simulink model "testemplannerglf_cs"  (R2020a)
settings: Solver=ode5  StartTime=0.0  StopTime=75  FixedStep=1/1000  RelTol=1e-3
PreLoadFcn:
  | mbxruntime.callbacks.PreLoadFcn(bdroot);
PostLoadFcn:
  | mbxruntime.callbacks.PostLoadFcn(bdroot);
InitFcn:
  | mbxruntime.callbacks.InitFcn(bdroot);
StartFcn:
  | mbxruntime.callbacks.StartFcn(bdroot);
StopFcn:
  | mbxruntime.callbacks.StopFcn(bdroot);
model workspace (MAT data in the model file):
  mbox_table : object (value not decoded)
  model_closed = 0
  sim_status = 0
values from neighbouring files (symbols this model uses):
  global_path_x = [-3.342 -2.8421723782 -2.34265574205 -1.8434543045 -1.34457058078 -0.846006057582 -0.347761597731 0.15016231435 0.647765423738 1.14504761469 1.64200885585 2.13864916705 ... (1501 elements, 1501x1)]    [global_path.mat]
  global_path_y = [4.7606 4.76495870158 4.76931469124 4.77366793224 4.77801840264 4.78236608949 4.78671098525 4.7910530857 4.79539238863 4.79972889301 4.80406259858 4.80839350551 ... (1501 elements, 1501x1)]    [global_path.mat]
undefined symbols (not defined in the file or in its folder): DiscIntNeverNeededParam, warningInitialVelocity, x0
libraries: simulink x19, PreScanSimulinkLibrary x11, simulink_extras x6, Solver_SF x1
(part 6 of 7)

== matlab function testemplannerglf_cs/Audi_A8_Sedan_1/decesion&&planning/referenceline provider/calc_heading_kappa1 ==
  data: path_x input; frenet_heading output; path_y input; frenet_kappa output
function [frenet_heading,frenet_kappa] = fcn(path_x,path_y)
%功能：该函数是利用已知的路径点计算heading和Kappa的值
%输入：path_x，path_y，全局路径点
%输出：frenet_heading，kappa
%2022 0310 glf 于寝室302

%注意事项，这里要注意角度的多值性，
%计算kappa时，kappa = dheading/ds，如果dheading差pi时tan值相等
%x和x+2pi往往代表同一个角度，但是（0.1-（-0.1））/ds和（0.1-（-0.1+2*pi））/ds差距较大
dx = diff(path_x);
dy = diff(path_y);

dx_pre = [dx(1);dx];
dx_after = [dx;dx(end)];
dx_final = (dx_pre + dx_after) / 2;

dy_pre = [dy(1);dy];
dy_after = [dy;dy(end)];
dy_final = (dy_pre + dy_after) / 2;

frenet_heading = atan2(dy_final,dx_final);

ds = sqrt(dx_final.^2 + dy_final.^2);
dheading = diff(frenet_heading);
dheading_pre = [dheading(1);dheading];
dheading_after = [dheading;dheading(end)];
dheading_final = (dheading_pre + dheading_after) / 2;

%为了防止dheading出现多了一个2pi的错误，假设真实的dheading较小，用sin（dheading）近似dheading
frenet_kappa = sin(dheading_final). / ds;

== matlab function testemplannerglf_cs/Audi_A8_Sedan_2/PathFollower_Preview_1/LateralController/Calculate delta steering error/eml_delta_steering_error ==
  data: v_x_vehicle input; v_x_vehicle_Min input; t_Preview_LatCtrl input; delta_steeringwheeltotal output; v_y_vehicle input; yawrate_vehicle input; CorneringStiffness_Tyres_Front input; CorneringStiffness_Tyres_Rear input; m_vehicle_total input; inertia_z_vehicle_total input; e_Lat input size=10; Pos_x_CoG_Vehicle input; wheelbase input; RefreshCounter parameter
function delta_steeringwheeltotal = eml_delta_steering_error(v_x_vehicle,v_x_vehicle_Min,t_Preview_LatCtrl,v_y_vehicle,yawrate_vehicle,CorneringStiffness_Tyres_Front,CorneringStiffness_Tyres_Rear,m_vehicle_total,inertia_z_vehicle_total,e_Lat,Pos_x_CoG_Vehicle,wheelbase,RefreshCounter)

delta_steeringwheeltotal = emlfcn_delta_steering_error(v_x_vehicle,v_x_vehicle_Min,t_Preview_LatCtrl,v_y_vehicle,yawrate_vehicle,CorneringStiffness_Tyres_Front,CorneringStiffness_Tyres_Rear,m_vehicle_total,inertia_z_vehicle_total,e_Lat,Pos_x_CoG_Vehicle,wheelbase,RefreshCounter);

% end function

== matlab function testemplannerglf_cs/Audi_A8_Sedan_1/decesion&&planning/emplanner planner/plan_start&&switch_trajectory ==
  data: pre_trajectory_x input; pre_trajectory_y input; pre_trajectory_heading input; pre_trajectory_kappa input; pre_trajectory_velocity input; pre_trajectory_accel input; pre_trajectory_time input; current_time input; host_x input; host_y input; host_heading_xy input; host_vx input; host_vy input; host_ax input; host_ay input; plan_start_x output; plan_start_y output; plan_start_heading output; plan_start_kappa output; plan_start_vx output; plan_start_vy output; plan_start_ax output; plan_start_ay output; plan_start_time output; switch_x output; switch_y output; switch_heading output; switch_kappa output; switch_speed output; switch_accel output; switch_time output
function [plan_start_x,plan_start_y,plan_start_heading,plan_start_kappa,plan_start_vx,plan_start_vy,plan_start_ax,plan_start_ay,plan_start_time,...
    switch_x,switch_y,switch_heading,switch_kappa,switch_speed,switch_accel,switch_time] = fcn(pre_trajectory_x,pre_trajectory_y,pre_trajectory_heading,...
    pre_trajectory_kappa,pre_trajectory_velocity,pre_trajectory_accel,pre_trajectory_time,current_time,host_x,host_y,host_heading_xy,host_vx,host_vy,host_ax,host_ay)
%功能:该函数将提供规划起点，拼接轨迹的消息
%输入：
%上个轨迹点的信息pre_trajectory_x,pre_trajectory_y,pre_trajectory_heading，pre_trajectory_kappa,pre_trajectory_velocity,pre_trajectory_accel,pre_trajectory_time
%现在的时间：current_time
%定位消息：host_x,host_y,host_heading_xy,host_vx,host_vy,host_ax,host_ay
%输出：
%规划轨迹的消息：plan_start_x,plan_start_y,plan_start_heading,plan_start_kappa,plan_start_vx,plan_start_vy,plan_start_ax,plan_start_ay,plan_start_time
%拼接轨迹的消息：switch_x,switch_y,switch_heading,switch_kappa,switch_speed,switch_accel,switch_time

%20220312 glf写于寝室302
%对拼接的轨迹初始化
n = 20;
switch_x = zeros(n,1);
switch_y = zeros(n,1);
switch_heading = zeros(n,1);
switch_kappa = zeros(n,1);
switch_speed = zeros(n,1);
switch_accel = zeros(n,1);
switch_time = ones(n,1) * -1;
persistent isFirstRun;
if isempty(isFirstRun)
    %代码首次运行
    isFirstRun = 0;
    %首次运行车辆的速度为0，因此不需要车辆动力学进行外推
    plan_start_x = host_x;
    plan_start_y = host_y;
    plan_start_heading = host_heading_xy;
    plan_start_kappa = 0;
    plan_start_vx = 0;
    plan_start_vy = 0;
    plan_start_ax = 0;
    plan_start_ay = 0;
    plan_start_time = current_time+0.1;
else
    x_cur = host_x;
    y_cur = host_y;
    kappa_cur = 0;
    %将车辆坐标的速度转换为世界坐标系
    vx_cur = host_vx*cos(host_heading_xy) - host_vy*sin(host_heading_xy);
    vy_cur = host_vx*sin(host_heading_xy) + host_vy*cos(host_heading_xy);
    ax_cur = host_ax*cos(host_heading_xy) - host_ay*sin(host_heading_xy);
    ay_cur = host_ax*sin(host_heading_xy) + host_ay*cos(host_heading_xy);
    %规划周期
    dt = 0.1;
    %判断当前时间在上个轨迹的那个位置
    for i = 1:(length(pre_trajectory_time) - 1)
       if pre_trajectory_time(i) <= current_time && pre_trajectory_time(i+1) > current_time 
          break; 
       end
    end
    
    %计算横纵向误差判断控制是否控制的完美
    pre_desire_heading = pre_trajectory_heading(i);
    %切向量
    tor = [cos(pre_desire_heading);sin(pre_desire_heading)];
    %法向量
    nor = [-sin(pre_desire_heading);cos(pre_desire_heading)];
    %位失
    direction = [host_x;host_y] - [pre_trajectory_x(i);pre_trajectory_y(i)];
    %横向误差
    lat_err = abs(direction'*nor);
    %纵向误差
    lon_err = abs(direction'*tor);
    if (lon_err > 2.5 || lat_err > 0.5)
        %控制没跟上
        plan_start_x = x_cur + vx_cur*dt + 0.5*ax_cur*dt*dt;
        plan_start_y = y_cur + vy_cur*dt + 0.5*ay_cur*dt*dt;
        plan_start_vx = vx_cur + ax_cur * dt;
        plan_start_vy = vy_cur + ay_cur * dt;
        plan_start_ax = ax_cur;
        plan_start_ay = ay_cur;
        plan_start_heading = atan2(plan_start_vy,plan_start_vx);
        plan_start_kappa = kappa_cur;
        %规划起点是当前时间点+100ms
        plan_start_time = current_time + 0.1;
    else
        %控制能跟上
        for j = i:length(pre_trajectory_time)-1
           if pre_trajectory_time(j) <= current_time + 0.1 &&pre_trajectory_time(j+1) < current_time
              break; 
           end
        end
        plan_start_x = pre_trajectory_x(j);
        plan_start_y = pre_trajectory_y(j);
        plan_start_heading = pre_trajectory_heading(j);
        plan_start_kappa = pre_trajectory_kappa(j);
        plan_start_vx = pre_trajectory_velocity*cos(plan_start_heading);
        plan_start_vy = pre_trajectory_velocity*sin(plan_start_heading);
        %切向量和法向量
        tor = [cos(plan_start_heading);sin(plan_start_heading)];
        nor = [-sin(plan_start_heading);cos(plan_start_heading)];
        a_tor = pre_trajectory_accel(j)*tor;
        a_nor = pre_trajectory_velocity(j)^2*plan_start_kappa*nor;
        plan_start_ax = a_tor(1) + a_nor(1);
        plan_start_ay = a_tor(2) + a_nor(2);
        plan_start_time = pre_trajectory_time(j);
        
        %进行轨迹拼接
        %还有一个细节需要考虑，pre_trajectory x(j) y(j)...是规划的起点，那么在轨迹拼接时
        %需不需要在stitch_trajectory中把pre_trajectory x(j) y(j)...包含进去
        %答案是否定的，不应该包含进去，因为规划的起点在规划模块计算完成后的结果中包含，如果在拼接的时候
        %还要包含，那就等于规划起点包含了两次
        %除非本周期计算的轨迹不包含规划起点，那么stitch_trajectory可以包含规划起点
        %如果本周期计算的轨迹包含规划起点，那么stitch_trajectory不可以包含规划起点
        %我们选择规划包含起点，拼接不包含起点的做法
 
        %把起点去掉
        j = j - 1;
        if j > 19
            switch_x = pre_trajectory_x(j-19:j);
            switch_y = pre_trajectory_y(j-19:j);
            switch_heading = pre_trajectory_heading(j-19:j);
            switch_kappa = pre_trajectory_kappa(j-19:j);
            switch_speed = pre_trajectory_velocity(j-19:j);
            switch_accel = pre_trajectory_accel(j-19:j);
            switch_time = pre_trajectory_time(j-19:j);
            
        else
            switch_x(20-j+1:20) = pre_trajectory_x(1:j);
            switch_y(20-j+1:20) = pre_trajectory_y(1:j);
            switch_heading(20-j+1:20) = pre_trajectory_heading(1:j);
            switch_kappa(20-j+1:20) = pre_trajectory_kappa(1:j);
            switch_speed(20-j+1:20) = pre_trajectory_velocity(1:j);
            switch_accel(20-j+1:20) = pre_trajectory_accel(1:j);
            switch_time(20-j+1:20) = pre_trajectory_time(1:j);
        end
    end
end

== matlab function testemplannerglf_cs/Audi_A8_Sedan_1/decesion&&planning/emplanner planner/index2s_calc ==
  data: reference_x input; index2s output; reference_y input; origin_x input; origin_y input; origin_match_point_index input
function index2s = fcn(reference_x,reference_y,origin_x,origin_y,origin_match_point_index)
    %功能：此函数是为了计算参考线上所有点的索引所对应的长度关系
    %输入：
    %参考线坐标：reference_x,reference_y
    %匹配点坐标：origin_x,origin_y，匹配点索引：origin_match_point_index
    %输出：
    %index2s储存了181个点的长度

    %2022 0315  glf 写于国实507
    n = 181;%一共有181个点
    index2s = zeros(n,1);
    for i = 2:181
       index2s(i) = sqrt((reference_x(i) - reference_x(i - 1))^2 + (reference_y(i) - reference_y(i - 1))^2) + index2s(i-1); 
    end

    %将index2s转换为以投影点为坐标原点
    s0 = fcn1(index2s,reference_x,reference_y,origin_x,origin_y,origin_match_point_index);

    index2s = index2s - s0*ones(n,1);
end

function s = fcn1(index2s,reference_x,reference_y,proj_x,proj_y,proj_match_point_index)
    %判断投影点是在匹配点的前面还是后面
    vector_1 = [proj_x;proj_y] - [reference_x(proj_match_point_index);reference_y(proj_match_point_index)];
    if proj_match_point_index < length(reference_x)
        vector_2 = [reference_x(proj_match_point_index + 1);reference_y(proj_match_point_index + 1)] - [reference_x(proj_match_point_index);reference_y(proj_match_point_index)];
    else
        vector_2 = [reference_x(proj_match_point_index);reference_y(proj_match_point_index)] - [reference_x(proj_match_point_index - 1);reference_y(proj_match_point_index - 1)];
    end

    if vector_1' * vector_2 > 0
        %投影点在匹配点前边
        s = index2s(proj_match_point_index) + sqrt(vector_1' * vector_1);
    else
        %投影点在匹配点后边
        s = index2s(proj_match_point_index) - sqrt(vector_1' * vector_1);
    end

end

== matlab function testemplannerglf_cs/Audi_A8_Sedan_1/peception_module/MATLAB Function ==
  data: host_x input; obs_x_set_gcs output; host_y input; host_heading_xy input; obs_range input; obs_theta input; obs_velocity input; obs_velocity_heading input; obs_y_set_gcs output; obs_velocity_set_gcs output; obs_heading_set_gcs output
function [obs_x_set_gcs, obs_y_set_gcs, obs_velocity_set_gcs, obs_heading_set_gcs] = ...
    fcn(host_x, host_y, host_heading_xy, obs_range, obs_theta, obs_velocity, obs_velocity_heading)
%gcs 全局坐标系global coordinate system
%该函数是感知模块，输出障碍物的位置，速度大小，速度方向与世界坐标系x轴的夹角
%输入：定位信息host_x,host_y,host_heading_xy世界坐标系
%      障碍物在传感器坐标下的极坐标range，theta
%      障碍物的速度大小 velocity
%      障碍物的速度方向与x轴的夹角heading
%输出：障碍物在世界坐标系下的坐标x y v x与x轴的夹角heading
%      注意输出的heading是在障碍物的速度heading，不是障碍物的几何2heading

%传感器最多输出32个障碍物信息，但是事先不知道有多少个障碍物，需要做个缓存

%输出初始化
obs_x_set_gcs = ones(32,1) * nan;
obs_y_set_gcs = ones(32,1) * nan;
obs_velocity_set_gcs = ones(32,1) * nan;
obs_heading_set_gcs = ones(32,1) * nan;
%传感器极坐标的角度顺时针为正，世界坐标是逆时针为正
theta_transfer = -obs_theta * pi /180;
%velocity的方向是向北为0度，世界坐标系是以向东为0度
heading_transfer = (-obs_velocity_heading + 90 * ones(32,1)) * pi / 180;
%计算障碍物到传感器的x方向距离，y方向距离
x_transfer = obs_range.*cos(theta_transfer + host_heading_xy);
y_transfer = obs_range.*sin(theta_transfer + host_heading_xy);

%计算障碍物的世界坐标
for i = 1:32
    if obs_range(i) ~= 0
        obs_x_set_gcs(i) = x_transfer(i) + host_x + 2.17 * cos(host_heading_xy);
        obs_y_set_gcs(i) = y_transfer(i) + host_y + 2.17 * sin(host_heading_xy);
        obs_heading_set_gcs(i) = heading_transfer(i);
        obs_velocity_set_gcs(i) = obs_velocity(i);
    end
end

== matlab function testemplannerglf_cs/Audi_A8_Sedan_1/decesion&&planning/emplanner planner/start_project ==
  data: host_x input; match_point_index_set output; host_y input; frenet_x input; frenet_y input; frenet_heading input; frenet_kappa input; project_x_set output; project_y_set output; project_heading_set output; project_kappa_set output
function [match_point_index_set,project_x_set,project_y_set,project_heading_set,project_kappa_set] =...
    fcn(host_x,host_y,frenet_x,frenet_y,frenet_heading,frenet_kappa)
%功能：该函数是为了求投影点的x，y,heading,kappa值，其中分成了首次运行和非首次运行，非首次运行条件下可以利用上一个周期运行的结果加速运算
%输入：host_x,host_y,frenet_x,frenet_y,frenet_heading,frenet_kappa
%输出：match_point_index_set, project_x、y_set， project_heading_set,proj_kappa_set
%2022 0309 glf写于国实507

%输出初始化
n = 128;%128只是用来存储数据的，实际中只用了第一个点.之后可以试试如果n=1看看程序能不能运行！！！！！
match_point_index_set = ones(n,1) * nan;
project_x_set = ones(n,1) * nan;
project_y_set = ones(n,1) * nan;
project_heading_set = ones(n,1) * nan;
project_kappa_set = ones(n,1) * nan;

%声明持久变量
persistent isFirstRun;
persistent pre_match_point_index_set;
persistent pre_frenet_x_set;
persistent pre_frenet_y_set;
persistent pre_frenet_heading_set;
persistent pre_frenet_kappa_set;

if isempty(isFirstRun)
    isFirstRun = 0;
    pre_frenet_x_set = frenet_x;
    pre_frenet_y_set = frenet_y;
    pre_frenet_heading_set = frenet_heading;
    pre_frenet_kappa_set = frenet_kappa;
    %初始化match_point的结果
    pre_match_point_index_set = ones(n,1)*nan;
    
    for i = 1:length(host_x)
        if isnan(host_x(i))
           break; 
        end
        start_index = 1;
        min_distance = inf;
        increase_count = 0;
        for j = start_index:length(frenet_x)
            distance = sqrt((host_x(i) - frenet_x(j))^2 + (host_y(i) - frenet_y(j))^2);
            if distance < min_distance
               distance = min_distance;
               match_point_index_set(i) = j;
            else
                increase_count = increase_count + 1;
            end
            if increase_count == 50
               break; 
            end
        end
        
        %由匹配点求投影点
        match_point_index = match_point_index_set(i);
        match_point_index_x = pre_frenet_x_set(match_point_index);%这里源代码写的是frenet_path_x
        match_point_index_y = pre_frenet_y_set(match_point_index);
        %匹配点位失
        match_point_direction = [match_point_index_x;match_point_index_y];
        %带投影点位失
        host_direction = [host_x;host_y];
        match_point_index_heading = pre_frenet_heading_set(match_point_index);
        match_point_index_kappa = pre_frenet_kappa_set(match_point_index);
        ds = (host_direction - match_point_direction)'*[cos(match_point_index_heading);sin(match_point_index_heading)];
        proj_index_set = match_point_direction + ds*[cos(match_point_index_heading);sin(match_point_index_heading)];
        proj_index_heading = match_point_index_heading + ds * match_point_index_kappa;
        proj_index_kappa = match_point_index_kappa;
        
        %输出计算结果
        project_x_set(i) = proj_index_set(1);
        project_y_set(i) = proj_index_set(2);
        project_heading_set(i) = proj_index_heading;
        project_kappa_set(i) = proj_index_kappa;   
    end
    pre_match_point_index_set = match_point_index_set;
    
else
    for i = 1:length(host_x)
        
        start_index = pre_match_point_index_set(i);
        %以下判断语句是为了防止感知时出现bug，具体还不懂
        %声明increase_count_limit
        increase_count_limit = 5;
        if isnan(start_search_index)
            increase_count_limit = 50;
            %搜索起点设为1
            start_search_index = 1;            
        end
        increase_count = 0; 
        
        %由上一个匹配点计算车辆的行驶方向
        %匹配点位失
        vector_match_point_index = [pre_frenet_x_set(start_index);pre_frenet_y_set(start_index)];
        %待投影点位失
        vector_host_point_index = [host_x;host_y];
        match_point_index_heading = pre_frenet_heading_set(start_index);
        flag = (vector_host_point_index - vector_match_point_index)'*[cos(match_point_index_heading);sin(match_point_index_heading)];
        if flag > 0.001
            min_distance = inf;
            for j = start_index:length(frenet_x)
                distance = sqrt((host_x(i) - frenet_x(j))^2 + (host_y(i) - frenet_y(j))^2);
                if distance < min_distance
                   distance = min_distance;
                   match_point_index_set(i) = j;
                else
                    increase_count = increase_count + 1;
                end
                if increase_count == increase_count_limit
                   break; 
                end
            end
        elseif flag < -0.001
            min_distance = inf;
            for j = start_index:-1:1
                distance = sqrt((host_x(i) - frenet_x(j))^2 + (host_y(i) - frenet_y(j))^2);
                if distance < min_distance
                   distance = min_distance;
                   match_point_index_set(i) = j;
                else
                    increase_count = increase_count + 1;
                end
                if increase_count == increase_count_limit
                   break; 
                end
            end
        else
            match_point_index_set(i) = start_index;
        end
        
        %由匹配点求投影点
        match_point_index = match_point_index_set(i);
        match_point_index_x = pre_frenet_x_set(match_point_index);%这里源代码写的是frenet_path_x
        match_point_index_y = pre_frenet_y_set(match_point_index);
        %匹配点位失
        match_point_direction = [match_point_index_x;match_point_index_y];
        %带投影点位失
        host_direction = [host_x;host_y];
        match_point_index_heading = pre_frenet_heading_set(match_point_index);
        match_point_index_kappa = pre_frenet_kappa_set(match_point_index);
        ds = (host_direction - match_point_direction)'*[cos(match_point_index_heading);sin(match_point_index_heading)];
        proj_index_set = match_point_direction + ds*[cos(match_point_index_heading);sin(match_point_index_heading)];
        proj_index_heading = match_point_index_heading + ds * match_point_index_kappa;
        proj_index_kappa = match_point_index_kappa;
        
        %输出计算结果
        project_x_set(i) = proj_index_set(1);
        project_y_set(i) = proj_index_set(2);
        project_heading_set(i) = proj_index_heading;
        project_kappa_set(i) = proj_index_kappa; 
    end
    pre_frenet_x_set = frenet_x;
    pre_frenet_y_set = frenet_y;
    pre_frenet_heading_set = frenet_heading;
    pre_frenet_kappa_set = frenet_kappa;
    pre_match_point_index_set = match_point_index_set;
end

== matlab function testemplannerglf_cs/Audi_A8_Sedan_1/decesion&&planning/emplanner planner/cattesian2Frenet/s&&l_calc ==
  data: x_set input; s_set output; y_set input; frenet_x_set input; frenet_y_set input; proj_x_set input; proj_y_set input; proj_heading_set input; proj_match_point_index input; l_set output; index2s input
function [s_set,l_set] = fcn(x_set,y_set, frenet_x_set,frenet_y_set,proj_x_set,proj_y_set,proj_heading_set,proj_match_point_index,index2s)
%功能：该函数是将规划起点时投影点从世界坐标系转换为frenet坐标下的s、l
%输入：x_set,y_set:规划开始的点的x和y坐标
%     frenet_x_set,frenet_y_set参考线的x、y坐标
%     proj_heading_set投影点的航向角 proj_match_point_index ：投影点匹配点索引
%     index2s：s的索引和长度的关系,这种算法加速了计算速度缩短了时间
%输出：s_set，l_set：frenet坐标下的s和l坐标

%2022 0317   glf 写于国实507
    %输出初始化
    n = 128;
    s_set = ones(n,1)*nan;
    l_set = ones(n,1)*nan;
    for i = 1:length(x_set)
        if isnan(x_set(i))
           break; 
        end
        s_set(i) = clacSFromIndex2s(index2s,frenet_x_set,frenet_y_set,proj_x_set(i),proj_y_set(i),proj_match_point_index(i));
        n_r = [-sin(proj_heading_set(i));cos(proj_heading_set(i))];
        r_h = [x_set(i);y_set(i)];
        r_r = [proj_x_set(i);proj_y_set(i)];
        l_set(i) = (r_h - r_r)'*n_r;
    end
    
end
function s = clacSFromIndex2s(index2s,frenet_x_set,frenet_y_set,proj_x_set,proj_y_set,proj_match_point_index)
    %判断投影点是在匹配点的前面还是后面
    vector_1 = [proj_x_set;proj_y_set] - [frenet_x_set(proj_match_point_index);frenet_y_set(proj_match_point_index)];
    if proj_match_point_index < length(reference_x)
        vector_2 = [frenet_x_set(proj_match_point_index + 1);frenet_y_set(proj_match_point_index + 1)] - [frenet_x_set(proj_match_point_index);frenet_y_set(proj_match_point_index)];
    else
        vector_2 = [frenet_x_set(proj_match_point_index);frenet_y_set(proj_match_point_index)] - [frenet_x_set(proj_match_point_index - 1);frenet_y_set(proj_match_point_index - 1)];
    end

    if vector_1' * vector_2 > 0
        %投影点在匹配点前边
        s = index2s(proj_match_point_index) + sqrt(vector_1' * vector_1);
    else
        %投影点在匹配点后边
        s = index2s(proj_match_point_index) - sqrt(vector_1' * vector_1);
    end
end

== matlab function testemplannerglf_cs/Audi_A8_Sedan_1/decesion&&planning/emplanner planner/cattesian2Frenet/s_dot&&l_dot&&dl_calc ==
  data: l_set input; s_dot_set output; vx_set input; vy_set input; proj_heading_set input; proj_kappa_set input; l_dot_set output; dl_set output
function [s_dot_set,l_dot_set,dl_set] = fcn(l_set,vx_set,vy_set,proj_heading_set,proj_kappa_set)
%功能：此函数功能是为了计算由世界坐标系转换为极坐标系下的s_dot, l_dot, dl_set
%输入：l_set计算得到的l的坐标的集合
%      vx_set，vy_set：世界坐标系的速度
%      proj_heading_set投影点的航向角   proj_kappa_set投影点的曲率
%输出：s_dot_set,l_dot_set,dl_set 坐标转换后的结果

%2022 0317  glf  写于国实507
%输出初始化
n = 128;
s_dot_set = ones(n,1)*nan;
l_dot_set = ones(n,1)*nan;
dl_set = ones(n,1)*nan;

for i = 1:length(l_set)
    if isnan(l_set(i))
       break;
    end
    v_h = [vx_set(i);vy_set(i)];
    t_r = [cos(proj_heading_set(i));sin(proj_heading_set(i))];
    n_r = [-sin(proj_heading_set(i));cos(proj_heading_set(i))];
    s_dot_set(i) = v_h' * t_r / (1 - proj_kappa_set(i)*l_set(i));
    
    l_dot_set(i) = v_h' * n_r;
    
    %利用向量法计算dl要避免速度为0的情况
    if s_dot_set(i) == 0
       dl_set(i) = 0; 
    else
        dl_set(i) = l_dot_set(i)/s_dot_set(i);
    end
end

== matlab function testemplannerglf_cs/Audi_A8_Sedan_1/decesion&&planning/emplanner planner/cattesian2Frenet/s_dot2&&l_dot2&&ddl_set_calc ==
  data: s_dot_set input; s_dot2_set output; l_set input; dl_set input; proj_heading_set input; proj_kappa_set input; ax_set input; ay_set input; l_dot2_set output; ddl_set output
function [s_dot2_set,l_dot2_set,ddl_set] = fcn(s_dot_set,l_set,dl_set,proj_heading_set,proj_kappa_set,ax_set,ay_set)
%功能：该函数是为了计算世界坐标系转换为frenet坐标系条件下的s_dot2_set,l_dot2_set,ddl_set
%输入：s_dot_set：坐标转换后的s_dot
%      l_set：frenet坐标系中的l坐标
%      dl_set坐标转换后的dl
%      proj_heading_set，proj_kappa_set投影点的航向角和曲率
%      ax_set，ay_set车辆的加速度
%输出：转换后的坐标系s_dot2_set,l_dot2_set,ddl_set

%2022 0317   glf 写于国实507

%输出初始化
n = 128;
s_dot2_set = ones(n,1);
l_dot2_set = ones(n,1);
ddl_set = ones(n,1);

for i = 1:length(l_set)
   if isnan(l_set(i))
      break; 
   end
   a_h = [ax_set(i);ay_set(i)];
   t_r = [cos(proj_heading_set(i));sin(proj_heading_set(i))];
   n_r = [-sin(proj_heading_set(i));cos(proj_heading_set(i))];
   
   l_dot2_set(i) = a_h' * n_r - proj_kappa_set(i)*(1 - proj_kappa_set(i) * l_set(i)) * (s_dot_set^2);
   %这里将dkr/ds设置为0，因为这个值极小，设置为0可以简化运算
   s_dot2_set(i) = 1/(1 - proj_kappa_set(i) * l_set(i)) * (a_h' * t_r + 2 * proj_kappa_set(i) * s_dot_set(i)^2 * l_set(i));
   %利用向量法计算时会出现速度为0的情况，因此分情况讨论
   if abs(s_dot_set(i)) < 1e-6
       ddl_set(i) = 0;
   else
       ddl_set(i) = (l_dot2_set(i) - dl_set(i) * s_dot2_set)/(s_dot_set(i)^2);
   end
   
end

== matlab function testemplannerglf_cs/Audi_A8_Sedan_1/decesion&&planning/emplanner planner/static_obs_filter/obs_cartesian2Frenetj/s&&l_calc ==
  data: x_set input; s_set output; y_set input; frenet_x_set input; frenet_y_set input; proj_x_set input; proj_y_set input; proj_heading_set input; proj_match_point_index input; l_set output; index2s input
function [s_set,l_set] = fcn(x_set,y_set, frenet_x_set,frenet_y_set,proj_x_set,proj_y_set,proj_heading_set,proj_match_point_index,index2s)
%功能：该函数是将规划起点时投影点从世界坐标系转换为frenet坐标下的s、l
%输入：x_set,y_set:规划开始的点的x和y坐标
%     frenet_x_set,frenet_y_set参考线的x、y坐标
%     proj_heading_set投影点的航向角 proj_match_point_index ：投影点匹配点索引
%     index2s：s的索引和长度的关系,这种算法加速了计算速度缩短了时间
%输出：s_set，l_set：frenet坐标下的s和l坐标

%2022 0317   glf 写于国实507
    %输出初始化
    n = 128;
    s_set = ones(n,1)*nan;
    l_set = ones(n,1)*nan;
    for i = 1:length(x_set)
        if isnan(x_set(i))
           break; 
        end
        s_set(i) = clacSFromIndex2s(index2s,frenet_x_set,frenet_y_set,proj_x_set(i),proj_y_set(i),proj_match_point_index(i));
        n_r = [-sin(proj_heading_set(i));cos(proj_heading_set(i))];
        r_h = [x_set(i);y_set(i)];
        r_r = [proj_x_set(i);proj_y_set(i)];
        l_set(i) = (r_h - r_r)'*n_r;
    end
    
end
function s = clacSFromIndex2s(index2s,frenet_x_set,frenet_y_set,proj_x_set,proj_y_set,proj_match_point_index)
    %判断投影点是在匹配点的前面还是后面
    vector_1 = [proj_x_set;proj_y_set] - [frenet_x_set(proj_match_point_index);frenet_y_set(proj_match_point_index)];
    if proj_match_point_index < length(reference_x)
        vector_2 = [frenet_x_set(proj_match_point_index + 1);frenet_y_set(proj_match_point_index + 1)] - [frenet_x_set(proj_match_point_index);frenet_y_set(proj_match_point_index)];
    else
        vector_2 = [frenet_x_set(proj_match_point_index);frenet_y_set(proj_match_point_index)] - [frenet_x_set(proj_match_point_index - 1);frenet_y_set(proj_match_point_index - 1)];
    end

    if vector_1' * vector_2 > 0
        %投影点在匹配点前边
        s = index2s(proj_match_point_index) + sqrt(vector_1' * vector_1);
    else
        %投影点在匹配点后边
        s = index2s(proj_match_point_index) - sqrt(vector_1' * vector_1);
    end
end

== matlab function testemplannerglf_cs/Audi_A8_Sedan_1/decesion&&planning/emplanner planner/static_obs_filter/obs_cartesian2Frenetj/s_dot&&l_dot&&dl_calc ==
  data: l_set input; s_dot_set output; vx_set input; vy_set input; proj_heading_set input; proj_kappa_set input; l_dot_set output; dl_set output
function [s_dot_set,l_dot_set,dl_set] = fcn(l_set,vx_set,vy_set,proj_heading_set,proj_kappa_set)
%功能：此函数功能是为了计算由世界坐标系转换为极坐标系下的s_dot, l_dot, dl_set
%输入：l_set计算得到的l的坐标的集合
%      vx_set，vy_set：世界坐标系的速度
%      proj_heading_set投影点的航向角   proj_kappa_set投影点的曲率
%输出：s_dot_set,l_dot_set,dl_set 坐标转换后的结果

%2022 0317  glf  写于国实507
%输出初始化
n = 128;
s_dot_set = ones(n,1)*nan;
l_dot_set = ones(n,1)*nan;
dl_set = ones(n,1)*nan;

for i = 1:length(l_set)
    if isnan(l_set(i))
       break;
    end
    v_h = [vx_set(i);vy_set(i)];
    t_r = [cos(proj_heading_set(i));sin(proj_heading_set(i))];
    n_r = [-sin(proj_heading_set(i));cos(proj_heading_set(i))];
    s_dot_set(i) = v_h' * t_r / (1 - proj_kappa_set(i)*l_set(i));
    
    l_dot_set(i) = v_h' * n_r;
    
    %利用向量法计算dl要避免速度为0的情况
    if s_dot_set(i) == 0
       dl_set(i) = 0; 
    else
        dl_set(i) = l_dot_set(i)/s_dot_set(i);
    end
end

== matlab function testemplannerglf_cs/Audi_A8_Sedan_1/decesion&&planning/emplanner planner/static_obs_filter/obs_cartesian2Frenetj/s_dot2&&l_dot2&&ddl_set_calc ==
  data: s_dot_set input; s_dot2_set output; l_set input; dl_set input; proj_heading_set input; proj_kappa_set input; ax_set input; ay_set input; l_dot2_set output; ddl_set output
function [s_dot2_set,l_dot2_set,ddl_set] = fcn(s_dot_set,l_set,dl_set,proj_heading_set,proj_kappa_set,ax_set,ay_set)
%功能：该函数是为了计算世界坐标系转换为frenet坐标系条件下的s_dot2_set,l_dot2_set,ddl_set
%输入：s_dot_set：坐标转换后的s_dot
%      l_set：frenet坐标系中的l坐标
%      dl_set坐标转换后的dl
%      proj_heading_set，proj_kappa_set投影点的航向角和曲率
%      ax_set，ay_set车辆的加速度
%输出：转换后的坐标系s_dot2_set,l_dot2_set,ddl_set

%2022 0317   glf 写于国实507

%输出初始化
n = 128;
s_dot2_set = ones(n,1);
l_dot2_set = ones(n,1);
ddl_set = ones(n,1);

for i = 1:length(l_set)
   if isnan(l_set(i))
      break; 
   end
   a_h = [ax_set(i);ay_set(i)];
   t_r = [cos(proj_heading_set(i));sin(proj_heading_set(i))];
   n_r = [-sin(proj_heading_set(i));cos(proj_heading_set(i))];
   
   l_dot2_set(i) = a_h' * n_r - proj_kappa_set(i)*(1 - proj_kappa_set(i) * l_set(i)) * (s_dot_set^2);
   %这里将dkr/ds设置为0，因为这个值极小，设置为0可以简化运算
   s_dot2_set(i) = 1/(1 - proj_kappa_set(i) * l_set(i)) * (a_h' * t_r + 2 * proj_kappa_set(i) * s_dot_set(i)^2 * l_set(i));
   %利用向量法计算时会出现速度为0的情况，因此分情况讨论
   if abs(s_dot_set(i)) < 1e-6
       ddl_set(i) = 0;
   else
       ddl_set(i) = (l_dot2_set(i) - dl_set(i) * s_dot2_set)/(s_dot_set(i)^2);
   end
   
end

== matlab function testemplannerglf_cs/Audi_A8_Sedan_1/decesion&&planning/emplanner planner/static_obs_filter/obs_filter ==
  data: host_x input; obs_x_set_final output; host_y input; host_heading_xy input; obs_x_set_gcs input; obs_y_set_gcs input; obs_y_set_final output; obs_velocity_set_final output; obs_heading_set_final output; obs_velocity_set_gcs input; obs_heading_set_gcs input
function [obs_x_set_final,obs_y_set_final,obs_velocity_set_final,obs_heading_set_final] = fcn(host_x,host_y,host_heading_xy,obs_x_set_gcs,obs_y_set_gcs,obs_velocity_set_gcs,obs_heading_set_gcs)
%功能：该函数是为了得到距离本车纵向距离为-10到60m，横向距离为-10到10m的障碍物的x，y坐标
%输入：host_x,host_y,host_heading_xy车辆的x，y坐标和航向角
%      obs_x_set_gcs,obs_y_set_gcs障碍物的x，y坐标
%输出：obs_x_set_final,obs_y_set_final在规定的范围内的障碍物的x，y坐标
%      obs_velocity_set_final,obs_heading_set_final障碍物的速度和航行角

%2022 0318   glf  写于国实507

%输出初始化,传感器最多可识别32个障碍物
n = 32;
obs_x_set_final = ones(n,1)*nan;
obs_y_set_final = ones(n,1)*nan;
obs_velocity_set_final = ones(n,1)*nan;
obs_heading_set_final = ones(n,1)*nan;

count = 1;
for i = 1:length(obs_x_set_gcs)
   if isnan(obs_x_set_gcs)
       break;
   end
   t_r = [cos(host_heading_xy);sin(host_heading_xy)];
   n_r = [-sin(host_heading_xy);cos(host_heading_xy)];
   %车辆到障碍物的向量
   v2obs_direction = [obs_x_set_gcs(i);obs_y_set_gcs(i)] - [host_x;host_y];
   lon_dis = v2obs_direction'*t_r;
   lat_dis = v2obs_direction'*n_r;
   %筛选障碍物
   if (lon_dis >= -10 && lon_dis < 60 && lat_dis >= -10 && lat_dis < 10)
      obs_x_set_final(count) = obs_x_set_gcs(i);
      obs_y_set_final(count) = obs_y_set_gcs(i);
      obs_velocity_set_final(count) = obs_velocity_set_gcs(i);
      obs_heading_set_final(count) = obs_heading_set_gcs(i);
      count = count + 1;
   end
end

== matlab function testemplannerglf_cs/Audi_A8_Sedan_1/decesion&&planning/emplanner planner/static_obs_filter/static_dynamic_filter ==
  data: obs_x_set_final input; obs_static_x_set output; obs_y_set_final input; obs_velocity_set_final input; obs_heading_set_final input; obs_static_y_set output; obs_dynamic_x_set output; obs_dynamic_y_set output; obs_dynamic_vx_set output; obs_dynamic_vy_set output
function [obs_static_x_set,obs_static_y_set,obs_dynamic_x_set,obs_dynamic_y_set,obs_dynamic_vx_set,obs_dynamic_vy_set] = ...
    fcn(obs_x_set_final,obs_y_set_final,obs_velocity_set_final,obs_heading_set_final)
%功能：该函数是为了区分静态障碍物和动态障碍物
%输入：obs_x_set_final,obs_y_set_final,obs_velocity_set_final,obs_heading_set_final障碍物对应的x，y坐标和速度、航向角
%输出：obs_static_x_set,obs_static_y_set 静态障碍物的x。y坐标
%     obs_dynamic_x_set,obs_dynamic_y_set,obs_dynamic_vx_set,obs_dynamic_vy_set动态障碍物的x，y坐标和vx、vy
%2022 0318     glf   写于国实507

%输出初始化，因为障碍物最多有32个
n = 32;
obs_static_x_set = ones(n,1)*nan;
obs_static_y_set = ones(n,1)*nan;
obs_dynamic_x_set = ones(n,1)*nan;
obs_dynamic_y_set = ones(n,1)*nan;
obs_dynamic_vx_set = ones(n,1)*nan;
obs_dynamic_vy_set = ones(n,1)*nan;

count_static = 1;
count_dynamic = 1;
for i = 1:length(obs_x_set_final)

    if abs(obs_velocity_set_final(i)) < 0.1%静态障碍物
        obs_static_x_set(count_static) = obs_x_set_final(i);
        obs_static_y_set(count_static) = obs_y_set_final(i);
        count_static = count_static + 1;
    else
        %动态障碍物
        obs_dynamic_x_set(count_dynamic) = obs_x_set_final(i);      
        obs_dynamic_y_set(count_dynamic) = obs_y_set_final(i);
        obs_dynamic_vx_set(count_dynamic) = obs_velocity_set_final(i)*cos(obs_heading_set_final(i));
        obs_dynamic_vy_set(count_dynamic) = obs_velocity_set_final(i)'*sin(obs_heading_set_final(i));
        count_dynamic = count_dynamic + 1;
    end
end

== matlab function testemplannerglf_cs/Audi_A8_Sedan_1/decesion&&planning/emplanner planner/static_obs_filter/obs_project ==
  data: host_x input; match_point_index_set output; host_y input; frenet_x input; frenet_y input; frenet_heading input; frenet_kappa input; project_x_set output; project_y_set output; project_heading_set output; project_kappa_set output
function [match_point_index_set,project_x_set,project_y_set,project_heading_set,project_kappa_set] =...
    fcn(host_x,host_y,frenet_x,frenet_y,frenet_heading,frenet_kappa)
%功能：该函数是为了求投影点的x，y,heading,kappa值，其中分成了首次运行和非首次运行，非首次运行条件下可以利用上一个周期运行的结果加速运算
%输入：host_x,host_y,frenet_x,frenet_y,frenet_heading,frenet_kappa
%输出：match_point_index_set, project_x、y_set， project_heading_set,proj_kappa_set
%2022 0309 glf写于国实507

%输出初始化
n = 128;%128只是用来存储数据的，实际中只用了第一个点.之后可以试试如果n=1看看程序能不能运行！！！！！
match_point_index_set = ones(n,1) * nan;
project_x_set = ones(n,1) * nan;
project_y_set = ones(n,1) * nan;
project_heading_set = ones(n,1) * nan;
project_kappa_set = ones(n,1) * nan;

%声明持久变量
persistent isFirstRun;
persistent pre_match_point_index_set;
persistent pre_frenet_x_set;
persistent pre_frenet_y_set;
persistent pre_frenet_heading_set;
persistent pre_frenet_kappa_set;

if isempty(isFirstRun)
    isFirstRun = 0;
    pre_frenet_x_set = frenet_x;
    pre_frenet_y_set = frenet_y;
    pre_frenet_heading_set = frenet_heading;
    pre_frenet_kappa_set = frenet_kappa;
    %初始化match_point的结果
    pre_match_point_index_set = ones(n,1)*nan;
    
    for i = 1:length(host_x)
        if isnan(host_x(i))
           break; 
        end
        start_index = 1;
        min_distance = inf;
        increase_count = 0;
        for j = start_index:length(frenet_x)
            distance = sqrt((host_x(i) - frenet_x(j))^2 + (host_y(i) - frenet_y(j))^2);
            if distance < min_distance
               distance = min_distance;
               match_point_index_set(i) = j;
            else
                increase_count = increase_count + 1;
            end
            if increase_count == 50
               break; 
            end
        end
        
        %由匹配点求投影点
        match_point_index = match_point_index_set(i);
        match_point_index_x = pre_frenet_x_set(match_point_index);%这里源代码写的是frenet_path_x
        match_point_index_y = pre_frenet_y_set(match_point_index);
        %匹配点位失
        match_point_direction = [match_point_index_x;match_point_index_y];
        %带投影点位失
        host_direction = [host_x;host_y];
        match_point_index_heading = pre_frenet_heading_set(match_point_index);
        match_point_index_kappa = pre_frenet_kappa_set(match_point_index);
        ds = (host_direction - match_point_direction)'*[cos(match_point_index_heading);sin(match_point_index_heading)];
        proj_index_set = match_point_direction + ds*[cos(match_point_index_heading);sin(match_point_index_heading)];
        proj_index_heading = match_point_index_heading + ds * match_point_index_kappa;
        proj_index_kappa = match_point_index_kappa;
        
        %输出计算结果
        project_x_set(i) = proj_index_set(1);
        project_y_set(i) = proj_index_set(2);
        project_heading_set(i) = proj_index_heading;
        project_kappa_set(i) = proj_index_kappa;   
    end
    pre_match_point_index_set = match_point_index_set;
    
else
    for i = 1:length(host_x)
        
        start_index = pre_match_point_index_set(i);
        %以下判断语句是为了防止感知时出现bug，具体还不懂
        %声明increase_count_limit
        increase_count_limit = 5;
        if isnan(start_search_index)
            increase_count_limit = 50;
            %搜索起点设为1
            start_search_index = 1;            
        end
        increase_count = 0; 
        
        %由上一个匹配点计算车辆的行驶方向
        %匹配点位失
        vector_match_point_index = [pre_frenet_x_set(start_index);pre_frenet_y_set(start_index)];
        %待投影点位失
        vector_host_point_index = [host_x;host_y];
        match_point_index_heading = pre_frenet_heading_set(start_index);
        flag = (vector_host_point_index - vector_match_point_index)'*[cos(match_point_index_heading);sin(match_point_index_heading)];
        if flag > 0.001
            min_distance = inf;
            for j = start_index:length(frenet_x)
                distance = sqrt((host_x(i) - frenet_x(j))^2 + (host_y(i) - frenet_y(j))^2);
                if distance < min_distance
                   distance = min_distance;
                   match_point_index_set(i) = j;
                else
                    increase_count = increase_count + 1;
                end
                if increase_count == increase_count_limit
                   break; 
                end
            end
        elseif flag < -0.001
            min_distance = inf;
            for j = start_index:-1:1
                distance = sqrt((host_x(i) - frenet_x(j))^2 + (host_y(i) - frenet_y(j))^2);
                if distance < min_distance
                   distance = min_distance;
                   match_point_index_set(i) = j;
                else
                    increase_count = increase_count + 1;
                end
                if increase_count == increase_count_limit
                   break; 
                end
            end
        else
            match_point_index_set(i) = start_index;
        end
        
        %由匹配点求投影点
        match_point_index = match_point_index_set(i);
        match_point_index_x = pre_frenet_x_set(match_point_index);%这里源代码写的是frenet_path_x
        match_point_index_y = pre_frenet_y_set(match_point_index);
        %匹配点位失
        match_point_direction = [match_point_index_x;match_point_index_y];
        %带投影点位失
        host_direction = [host_x;host_y];
        match_point_index_heading = pre_frenet_heading_set(match_point_index);
        match_point_index_kappa = pre_frenet_kappa_set(match_point_index);
        ds = (host_direction - match_point_direction)'*[cos(match_point_index_heading);sin(match_point_index_heading)];
        proj_index_set = match_point_direction + ds*[cos(match_point_index_heading);sin(match_point_index_heading)];
        proj_index_heading = match_point_index_heading + ds * match_point_index_kappa;
        proj_index_kappa = match_point_index_kappa;
        
        %输出计算结果
        project_x_set(i) = proj_index_set(1);
        project_y_set(i) = proj_index_set(2);
        project_heading_set(i) = proj_index_heading;
        project_kappa_set(i) = proj_index_kappa; 
    end
    pre_frenet_x_set = frenet_x;
    pre_frenet_y_set = frenet_y;
    pre_frenet_heading_set = frenet_heading;
    pre_frenet_kappa_set = frenet_kappa;
    pre_match_point_index_set = match_point_index_set;
end

== matlab function testemplannerglf_cs/Audi_A8_Sedan_1/decesion&&planning/emplanner planner/dynamic_plan ==
  data: obs_s_set input; obs_l_set input; plan_start_s input; plan_start_l input; plan_start_dl input; plan_start_dll input; w_cost_collision input; w_cost_smooth_dl input; w_cost_smooth_ddl input; w_cost_smooth_dddl input; w_cost_ref input; row input; col input; sample_s input; sample_l input; dp_path_s output; dp_path_l output
function [dp_path_s,dp_path_l] = fcn(obs_s_set,obs_l_set,plan_start_s,plan_start_l,plan_start_dl,plan_start_dll,...
    w_cost_collision,w_cost_smooth_dl,w_cost_smooth_ddl,w_cost_smooth_dddl,w_cost_ref,row,col,sample_s,sample_l)

%动态规划的代码，用于寻找粗解，寻找最小代价的节点
node_cost = ones(row,col)*inf;
%初始化上一个节点的行的矩阵
pre_node_index = zeros(row,col);
%计算第一层
for i = 1:row
   node_cost(i,1) = costfirstlayer(plan_start_s,plan_start_l,plan_start_dl,plan_start_dll,...
    w_cost_collision,w_cost_smooth_dl,w_cost_smooth_ddl,w_cost_smooth_dddl,w_cost_ref,i,sample_s,sample_l,obs_s_set,obs_l_set); 
end

for j = 2:col
    for i = 1:row
        cur_node_s = plan_start_s + (j - 1)*sample_s;
        cur_node_l = ((row+1)/2 - i) * sample_l;
        %遍历前一列的节点
        for k = 1:row
            pre_node_s = plan_start_s + (j - 2)*sample_s;
            pre_node_l = ((row-1)/2 - k) * sample_l;
            cost_Neighbour = costNeighbour(pre_node_s,pre_node_l,cur_node_s,cur_node_l,w_cost_collision,...
                                w_cost_smooth_dl,w_cost_smooth_ddl,w_cost_smooth_dddl,w_cost_ref,obs_s_set,obs_l_set);
            cost_temp = node_cost(k,j-1) + cost_Neighbour;
            if cost_temp < node_cost(i,j)
                node_cost(i,j) = cost_temp;
                %保存下最小的节点的行号
                pre_node_index(i,j) = k;
            end
        end
    end
end

%找到node_cost中最后一列最小代价的cost,记代价最小的行为Index
index = 0;
node_cost_final = inf;
for i = 1:row
   if node_cost(i,end) < node_cost_final
      node_cost_final = node_cost(i,end);
      index = i;
   end
end

%倒推最小路径所在的所有节点
dp_node_list_row = zeros(col,1);
cur_index = index;
for i = 1:col
   pre_index = pre_node_index(cur_index,end-i+1); 
   dp_node_list_row(end-i+1) = cur_index;
   cur_index = pre_index;
end

%由于不知道有多少点，所以在这里要做个缓冲
dp_path_s = zeros(15,1);
dp_path_l = zeros(15,1);

for i = 1:col
   dp_path_s(i) = plan_start_s + (i-1)*sample_s;
   dp_path_l(i) = ((row + 1)/2 - dp_node_list_row(i))*sample_l;
end

end

function cost_Neighbour = costNeighbour(pre_node_s,pre_node_l,cur_node_s,cur_node_l,w_cost_collision,...
                                w_cost_smooth_dl,w_cost_smooth_ddl,w_cost_smooth_dddl,w_cost_ref,obs_s_set,obs_l_set)
   start_l = pre_node_l;
   start_dl = 0;
   start_ddl = 0;
   end_l = cur_node_l;
   end_dl = 0;
   end_ddl = 0;
   start_s = pre_node_s;
   end_s = cur_node_s;
   
   coeff = CalcQuinticCoefficient(start_l,start_dl,start_ddl,end_l,end_dl,end_ddl,start_s,end_s);
   a0 = coeff(1);
   a1 = coeff(2);
   a2 = coeff(3);
   a3 = coeff(4);
   a4 = coeff(5);
   a5 = coeff(6);
   %取十个点计算代价
   l= zeros(10,1);
   ds = zeros(10,1);
   dl = zeros(10,1);
   ddl = zeros(10,1);
   dddl = zeros(10,1);
   for i = 1:10
       ds(i) = start_s + (i-1)*sample_s/10;
   end
   l = a0 + a1*ds + a2*ds.^2 + a3*ds.^3 + a4*ds.^4 + a5*ds.^5;
   dl = a1 + 2*a2*ds + 3*a3*ds.^2 + 4*a4*ds.^3 + 5*a5*ds.^4;
   ddl = 2*a2 + 6*a3*ds + 12*a4*ds.^2 + 20*a5*ds.^3;
   dddl = 2 + 6*a3 + 24*a4*ds + 60*a5*ds.^2;
   cost_smooth = w_cost_smooth_dl*(dl'*dl) + w_cost_smooth_ddl*(ddl'*ddl) + w_cost_smooth_dddl*(dddl'*dddl);
   cost_ref = w_cost_ref*l'*l;
   cost_collision = 0;
   for i = 1:length(obs_s_set)
      if isnan(obs_s_set(i))
          break;
      end
      dlon = ones(10,1)*obs_s_set(i) - ds;
      dlat = ones(10,1)*obs_l_set(i) - l;
      squared_d = dlon.^2 + dlat.^2;
      cost_collison_temp = CalcObsCost(w_cost_collision,squared_d);
      cost_collision = cost_collison_temp + cost_collision;
   end
   cost_Neighbour = cost_smooth + cost_ref + cost_collision;
end
                            
function cost = costfirstlayer(begin_s,begin_l,begin_dl,begin_ddl,cur_node_row,sample_s,sample_l,w_cost_collision,...
    w_cost_smooth_dl,w_cost_smooth_ddl,w_cost_smooth_dddl,w_cost_ref,obs_s_set,obs_l_set)
   start_l = begin_l;
   start_dl = begin_dl;
   start_ddl = begin_ddl;
   
   end_l = (((row + 1)/2) - cur_node_row) * sample_l;
   end_dl = 0;
   end_ddl = 0;
   start_s = begin_s;
   end_s = start_s + sample_s;
   
   coeff = CalcQuinticCoefficient(start_l,start_dl,start_ddl,end_l,end_dl,end_ddl,start_s,end_s);
   a0 = coeff(1);
   a1 = coeff(2);
   a2 = coeff(3);
   a3 = coeff(4);
   a4 = coeff(5);
   a5 = coeff(6);
   %取十个点计算代价
   l= zeros(10,1);
   ds = zeros(10,1);
   dl = zeros(10,1);
   ddl = zeros(10,1);
   dddl = zeros(10,1);
   for i = 1:10
       ds(i) = start_s + (i-1)*sample_s/10;
   end
   l = a0 + a1*ds + a2*ds.^2 + a3*ds.^3 + a4*ds.^4 + a5*ds.^5;
   dl = a1 + 2*a2*ds + 3*a3*ds.^2 + 4*a4*ds.^3 + 5*a5*ds.^4;
   ddl = 2*a2 + 6*a3*ds + 12*a4*ds.^2 + 20*a5*ds.^3;
   dddl = 2 + 6*a3 + 24*a4*ds + 60*a5*ds.^2;
   cost_smooth = w_cost_smooth_dl*(dl'*dl) + w_cost_smooth_ddl*(ddl'*ddl) + w_cost_smooth_dddl*(dddl'*dddl);
   cost_ref = w_cost_ref*l'*l;
   cost_collision = 0;
   for i = 1:length(obs_s_set)
      if isnan(obs_s_set(i))
          break;
      end
      dlon = ones(10,1)*obs_s_set(i) - ds;
      dlat = ones(10,1)*obs_l_set(i) - l;
      squared_d = dlon.^2 + dlat.^2;
      cost_collison_temp = CalcObsCost(w_cost_collision,squared_d);
      cost_collision = cost_collison_temp + cost_collision;
   end
   cost = cost_smooth + cost_ref + cost_collision;
   
end

function obs_cost = CalcObsCost(w_cost_collision,squared_d)
    cost = 0;
    for i = 1:length(squared_d)
        if squared_d <9
            cost = cost + w_cost_collision;
        elseif squared_d >= 9 && squared_d < 16
            cost = cost + 1000/squared_d(i);
        end
    end
    obs_cost = cost;
end

function coeff = CalcQuinticCoefficient(start_l,start_dl,start_ddl,end_l,end_dl,end_ddl,start_s,end_s)
   start_s2 = start_s * start_s;
   start_s3 = start_s2 * start_s;
   start_s4 = start_s3 * start_s;
   start_s5 = start_s4 * start_s;
   
   end_s2 = end_s * end_s;
   end_s3 = end_s2 * end_s;
   end_s4 = end_s3 * end_s;
   end_s5 = end_s4 * end_s;
   A = [0,start_s, start_s2, start_s3,  start_s4,   start_s5;
        0,0,       2*start_s,3*start_s2,4*start_s3, 5*start_s4;
        0,0,       0,        6*start_s, 12*start_s2,20*start_s3;
        0,end_s, end_s2, end_s3,  end_s4,   end_s5;
        0,0,     2*end_s,3*end_s2,4*end_s3, 5*end_s4;
        0,0,     0,      6*end_s, 12*end_s2,20*end_s3;];
    B = [start_l;
        start_dl;
        start_ddl;
        end_l;
        end_dl;
        end_ddl;];
    coeff = A\B;

end
